simulink model "saved3"  (R2018b)
settings: Solver=VariableStepAuto  StartTime=0.0  StopTime=10.0  RelTol=1e-3
libraries: simulink x95, powerlib x8, powerlib_meascontrol x2
(part 1 of 6)
settings Model: Creator=71873  LastModifiedBy=71873

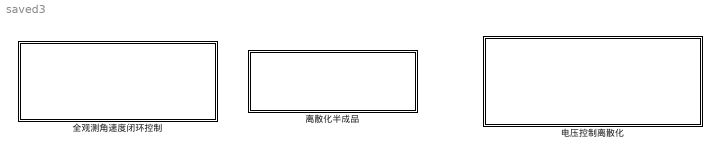
== system saved3 ==
  全观测角速度闭环控制 : Subsystem
  电压控制离散化 : Subsystem
  离散化半成品 : Subsystem

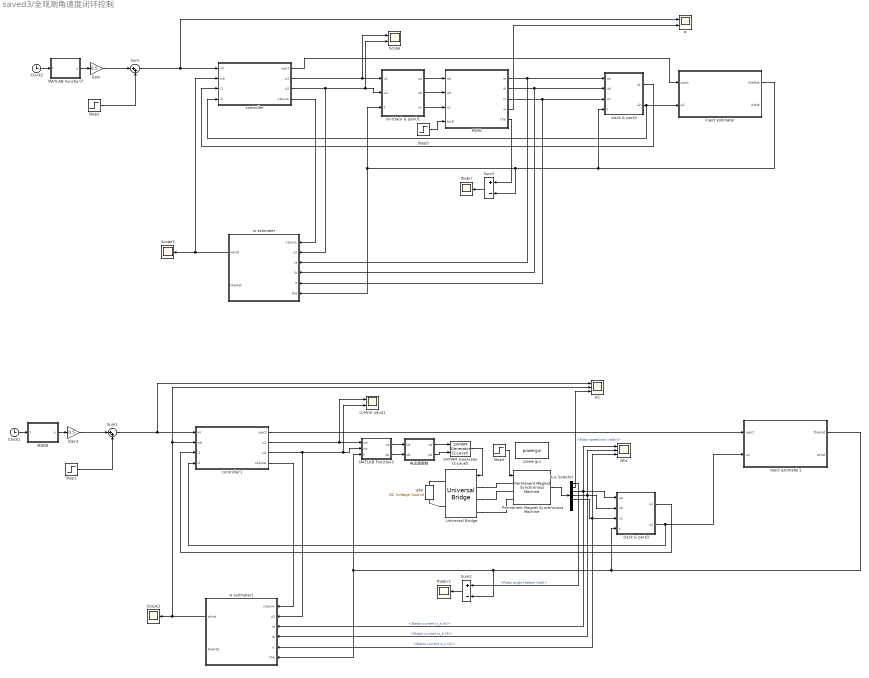
== system saved3/全观测角速度闭环控制 ==
  24V : powerlib/Electrical Sources/DC Voltage Source  Amplitude=24  Measurements=None
  Bus Selector : BusSelector  OutputSignals=Rotor angle thetam (rad),Rotor speed wm (rad/s),Stator current is_a (A),Stator current is_b (A),Stator current is_c (A),Stator current is_d (A),Stator current is_q (A)
  Clock1 : Clock
  Clock2 : Clock
  Gain : Gain  Gain=0.5
  Gain1 : Gain  Gain=0.5
  MATLAB Function3 : MATLAB Function  TreatAsAtomicUnit=on
  MATLAB Function7 : MATLAB Function  TreatAsAtomicUnit=on
  PSMS : Subsystem
  Permanent Magnet Synchronous Machine : powerlib/Machines/Permanent Magnet Synchronous Machine  NbPhases=3  FluxDistribution=Sinusoidal  RotorType=Salient-pole  MechanicalLoad=Torque Tm  PresetModel=No  ShowDetailedParameters=on  MeasurementBus=off  Resistance=0.1  Inductance=8.5e-3  dqInductances=[1e-3,1.4e-3]  La=0.000395  MachineConstant=Flux linkage established by magnets (V.s)  Flux=0.05  VoltageCst=9.069  TorqueCst=0.075  Flat=120  Mechanical=[1e-3 5e-4 1 0]  PolePairs=4  InitialConditions=[0,0, 0,0]  InitialConditions5ph=[0 0 0 0 0 0]  TsPowergui=0  TsBlock=-1  RefAngle=Aligned with phase A axis (original Park)
      settings: SourceProductName=Simscape Power Systems
  SVPWM Generator (2-Level) : powerlib_meascontrol/Pulse & Signal Generators/SVPWM Generator (2-Level)  InputType=alpha-beta components  SwitchingPattern=Pattern #1  Fc=20000  ParUref=[0.8 -30 50]  Ts=0
      settings: SourceProductName=Simscape Power Systems  SourceProductBaseCode=PS
  Scope : Scope  NumInputPorts=2
  Scope1 : Scope
  Scope3 : Scope
  Step1 : Step  Time=1.5  After=50  SampleTime=0
  Step2 : Step  Time=1.5  After=50  SampleTime=0
  Step3 : Step  After=0.5  SampleTime=0
  Step5 : Step  Time=0.8  After=0.25  SampleTime=0
  Sum : Sum  Inputs=|++
  Sum1 : Sum  Inputs=|++
  Sum2 : Sum  Inputs=+-
  Sum3 : Sum  Inputs=+-
  Universal Bridge : powerlib/Power Electronics/Universal Bridge  Arms=3  SnubberResistance=1e5  SnubberCapacitance=inf  Device=MOSFET / Diodes  Ron=1e-3  Lon=0  ForwardVoltages="[  0  0  ]"  ForwardVoltage=0  GTOparameters=[ 10e-6 , 20e-6 ]  IGBTparameters=[ 1e-6 , 2e-6 ]  Measurements=None  Measurements_2=None  converterType=Rectifier
  clack & park2 : MATLAB Function  TreatAsAtomicUnit=on
  clack & park3 : MATLAB Function  TreatAsAtomicUnit=on
  control uduq1 : Scope  NumInputPorts=2
  controller : Subsystem
  controller1 : Subsystem
  iabc : Scope  NumInputPorts=3
  inject estimater : Subsystem
  inject estimater1 : Subsystem
  inv(clack & park)1 : MATLAB Function  TreatAsAtomicUnit=on
  powergui : powerlib/powergui  Priority=1  SimulationMode=Discrete  SampleTime=1e-6  frequency=60  Iterations=50  frequencyindice=0  Pbase=100e6  ErrMax=1e-4  UnitsV=kV  UnitsW=MW  buscounter=0  FunctionMessages=off  echomessages=off  EnableUseOfTLC=off  CurrentSourceSwitches=off  DisableSnubberDevices=off  DisableRonSwitches=off  DisableVfSwitches=off  DisplayEquations=off  SolverType=Tustin/Backward Euler (TBE)  Interpol=off  ExternalGateDelay=off  methode=off  Ts=100  x0status=blocks  SPID=on  SwTol=0  HookPort=off  RestoreLinks=warning  ResistiveCurrentMeasurement=off  Frange=[0:2:500]  Ylog=off  Xlog=on  ShowGrid=off  save=off  variable=ZData  structure=0  ZoomFFT=off  StartTime=0.0  cycles=1  DisplayStyle=1  fundamental=60  FreqAxis=off  MaxFrequency=1000  frequencyindicesteady=1  RmsSteady=1  display=off
  theErr : Scope
  theErr1 : Scope
  w : Scope  NumInputPorts=2
  w estimater : Subsystem
  w estimater1 : Subsystem
  w1 : Scope  NumInputPorts=3
  电压圆限制 : MATLAB Function  TreatAsAtomicUnit=on
  软启动 : MATLAB Function  TreatAsAtomicUnit=on
  wires:
  controller/3(u2) -> inv(clack & park)1/2(u2), Scope/2, w estimater/2(u2)
  controller/2(u1) -> Scope/1, inv(clack & park)1/1(u1)
  Clock2/1 -> MATLAB Function7/1(t)
  inv(clack & park)1/2(ub) -> PSMS/2(ub)
  PSMS/2(ib) -> clack & park2/2(ub), w estimater/4(ib)
  Gain/1 -> Sum/1
  controller/4(u1pure) -> w estimater/1(u1pure)
  PSMS/5(the) -> Sum3/1
  MATLAB Function7/1(y) -> Gain/1
  Sum3/1 -> theErr/1
  PSMS/3(ic) -> clack & park2/3(uc), w estimater/5(ic)
  Step3/1 -> PSMS/4(torE)
  clack & park2/1(u1) -> controller/3(i1)
  PSMS/4(w) -> w/2
  inject estimater/1(theHat) -> inv(clack & park)1/3(t), w estimater/6(the), Sum3/2, clack & park2/4(t)
  inv(clack & park)1/3(uc) -> PSMS/3(uc)
  controller/1(uject) -> inject estimater/1(uject)
  w estimater/1(wHat) -> controller/2(wb), Scope3/1
  Sum/1 -> w/1, controller/1(wr)
  clack & park2/2(u2) -> controller/4(i2), inject estimater/2(u2)
  Step2/1 -> Sum/2
  inv(clack & park)1/1(ua) -> PSMS/1(ua)
  PSMS/1(ia) -> clack & park2/1(ua), w estimater/3(ia)
  controller1/4(u1pure) -> w estimater1/1(u1pure)
  Clock1/1 -> 软启动/1(t)
  Sum2/1 -> theErr1/1
  controller1/1(uject) -> inject estimater1/1(uject)
  clack & park3/1(u1) -> controller1/3(i1)
  SVPWM Generator (2-Level)/1 -> Universal Bridge/1
  clack & park3/2(u2) -> inject estimater1/2(u2), controller1/4(i2)
  Bus Selector/1 -> Sum2/1  "<Rotor angle thetam (rad)>"
  Bus Selector/4 -> w estimater1/4(ib), iabc/2, clack & park3/2(ub)  "<Stator current is_b (A)>"
  软启动/1(y) -> Gain1/1
  Permanent Magnet Synchronous Machine/1 -> Bus Selector/1
  MATLAB Function3/2(ub) -> 电压圆限制/2(Ub)
  Step5/1 -> Permanent Magnet Synchronous Machine/1
  inject estimater1/1(theHat) -> clack & park3/4(t), MATLAB Function3/3(t), w estimater1/6(the), Sum2/2
  Bus Selector/3 -> w estimater1/3(ia), iabc/1, clack & park3/1(ua)  "<Stator current is_a (A)>"
  controller1/2(u1) -> MATLAB Function3/1(ud), control uduq1/1
  MATLAB Function3/1(ua) -> 电压圆限制/1(Ua)
  电压圆限制/2(ub) -> SVPWM Generator (2-Level)/2
  controller1/3(u2) -> MATLAB Function3/2(uq), control uduq1/2, w estimater1/2(u2)
  Step1/1 -> Sum1/2
  电压圆限制/1(ua) -> SVPWM Generator (2-Level)/1
  w estimater1/1(wHat) -> w1/2, controller1/2(wb), Scope1/1
  Bus Selector/5 -> w estimater1/5(ic), iabc/3, clack & park3/3(uc)  "<Stator current is_c (A)>"
  Gain1/1 -> Sum1/1
  Bus Selector/2 -> w1/3  "<Rotor speed wm (rad/s)>"
  Sum1/1 -> w1/1, controller1/1(wr)
  connections:
  Universal Bridge/LConn3 -- Permanent Magnet Synchronous Machine/LConn3
  Universal Bridge/RConn1 -- 24V/RConn1
  Universal Bridge/RConn2 -- 24V/LConn1
  Universal Bridge/LConn2 -- Permanent Magnet Synchronous Machine/LConn2
  Universal Bridge/LConn1 -- Permanent Magnet Synchronous Machine/LConn1

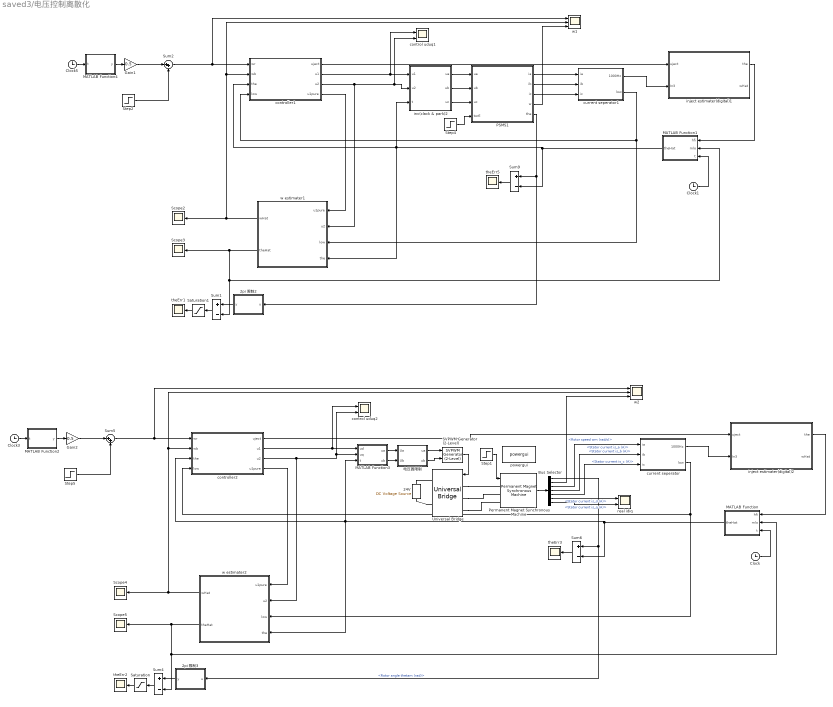
== system saved3/电压控制离散化 ==
  24V : powerlib/Electrical Sources/DC Voltage Source  Amplitude=24  Measurements=None
  2pi 限制2 : MATLAB Function  TreatAsAtomicUnit=on
  2pi 限制3 : MATLAB Function  TreatAsAtomicUnit=on
  Bus Selector : BusSelector  OutputSignals=Rotor angle thetam (rad),Rotor speed wm (rad/s),Stator current is_a (A),Stator current is_b (A),Stator current is_c (A),Stator current is_d (A),Stator current is_q (A)
  Clock{,1,3,5} (4 alike) : Clock
  Gain1 : Gain  Gain=0.5
  Gain2 : Gain  Gain=0.5
  MATLAB Function : MATLAB Function  TreatAsAtomicUnit=on
  MATLAB Function1 : MATLAB Function  TreatAsAtomicUnit=on
  MATLAB Function2 : MATLAB Function  TreatAsAtomicUnit=on
  MATLAB Function3 : MATLAB Function  TreatAsAtomicUnit=on
  MATLAB Function4 : MATLAB Function  TreatAsAtomicUnit=on
  PSMS1 : Subsystem
  Permanent Magnet Synchronous Machine : powerlib/Machines/Permanent Magnet Synchronous Machine  NbPhases=3  FluxDistribution=Sinusoidal  RotorType=Salient-pole  MechanicalLoad=Torque Tm  PresetModel=No  ShowDetailedParameters=on  MeasurementBus=off  Resistance=0.1  Inductance=8.5e-3  dqInductances=[1e-3,1.4e-3]  La=0.000395  MachineConstant=Flux linkage established by magnets (V.s)  Flux=0.05  VoltageCst=9.069  TorqueCst=0.075  Flat=120  Mechanical=[1e-3 5e-4 1 0]  PolePairs=4  InitialConditions=[0,0, 0,0]  InitialConditions5ph=[0 0 0 0 0 0]  TsPowergui=0  TsBlock=-1  RefAngle=Aligned with phase A axis (original Park)
      settings: SourceProductName=Simscape Power Systems
  SVPWM Generator (2-Level) : powerlib_meascontrol/Pulse & Signal Generators/SVPWM Generator (2-Level)  InputType=alpha-beta components  SwitchingPattern=Pattern #1  Fc=20000  ParUref=[0.8 -30 50]  Ts=0
      settings: SourceProductName=Simscape Power Systems  SourceProductBaseCode=PS
  Saturation : Saturate  UpperLimit=1  LowerLimit=-1
  Saturation1 : Saturate  UpperLimit=1  LowerLimit=-1
  Scope{2..5} (4 alike) : Scope
  Step1 : Step  Time=0.8  After=0.25  SampleTime=0
  Step2 : Step  Time=2  After=50  SampleTime=0
  Step4 : Step  After=0.5  SampleTime=0
  Step5 : Step  Time=2  After=50  SampleTime=0
  Sum{1,4,6,9} (4 alike) : Sum  Inputs=+-
  Sum2 : Sum  Inputs=|++
  Sum5 : Sum  Inputs=|++
  Universal Bridge : powerlib/Power Electronics/Universal Bridge  Arms=3  SnubberResistance=1e5  SnubberCapacitance=inf  Device=MOSFET / Diodes  Ron=1e-3  Lon=0  ForwardVoltages="[  0  0  ]"  ForwardVoltage=0  GTOparameters=[ 10e-6 , 20e-6 ]  IGBTparameters=[ 1e-6 , 2e-6 ]  Measurements=None  Measurements_2=None  converterType=Rectifier
  control uduq1 : Scope  NumInputPorts=2
  control uduq2 : Scope  NumInputPorts=2
  controller1 : Subsystem
  controller2 : Subsystem
  current seperator : Subsystem
  current seperator1 : Subsystem
  inject estimater(digital)1 : Subsystem
  inject estimater(digital)2 : Subsystem
  inv(clack & park)2 : MATLAB Function  TreatAsAtomicUnit=on
  powergui : powerlib/powergui  Priority=1  SimulationMode=Discrete  SampleTime=1e-6  frequency=60  Iterations=50  frequencyindice=0  Pbase=100e6  ErrMax=1e-4  UnitsV=kV  UnitsW=MW  buscounter=0  FunctionMessages=off  echomessages=off  EnableUseOfTLC=off  CurrentSourceSwitches=off  DisableSnubberDevices=off  DisableRonSwitches=off  DisableVfSwitches=off  DisplayEquations=off  SolverType=Tustin/Backward Euler (TBE)  Interpol=off  ExternalGateDelay=off  methode=off  Ts=100  x0status=blocks  SPID=on  SwTol=0  HookPort=off  RestoreLinks=warning  ResistiveCurrentMeasurement=off  Frange=[0:2:500]  Ylog=off  Xlog=on  ShowGrid=off  save=off  variable=ZData  structure=0  ZoomFFT=off  StartTime=0.0  cycles=1  DisplayStyle=1  fundamental=60  FreqAxis=off  MaxFrequency=1000  frequencyindicesteady=1  RmsSteady=1  display=off
  real idiq : Scope  NumInputPorts=2
  theErr{1..3,5} (4 alike) : Scope
  w estimater1 : Subsystem
  w estimater2 : Subsystem
  w1 : Scope  NumInputPorts=3
  w2 : Scope  NumInputPorts=3
  电压圆限制 : MATLAB Function  TreatAsAtomicUnit=on
  wires:
  controller2/2(u1) -> MATLAB Function3/1(ud), control uduq2/1
  电压圆限制/1(ua) -> SVPWM Generator (2-Level)/1
  w estimater2/1(wHat) -> Scope4/1, w2/2, controller2/2(wb)
  Bus Selector/6 -> real idiq/1  "<Stator current is_d (A)>"
  Clock3/1 -> MATLAB Function2/1(t)
  MATLAB Function2/1(y) -> Gain2/1
  Gain2/1 -> Sum5/1
  Saturation/1 -> theErr2/1
  w estimater2/2(theHat) -> Sum4/2, MATLAB Function/2(mlo), Scope5/1
  Sum4/1 -> Saturation/1
  Step1/1 -> Permanent Magnet Synchronous Machine/1
  Clock/1 -> MATLAB Function/3(t)
  Sum5/1 -> w2/1, controller2/1(wr)
  Step5/1 -> Sum5/2
  Bus Selector/5 -> current seperator/3(ic)  "<Stator current is_c (A)>"
  MATLAB Function3/2(ub) -> 电压圆限制/2(Ub)
  2pi 限制3/1(y) -> Sum4/1
  MATLAB Function/1(theHat) -> controller2/3(the), w estimater2/4(the), MATLAB Function3/3(t), Sum6/2
  Sum6/1 -> theErr3/1
  Permanent Magnet Synchronous Machine/1 -> Bus Selector/1
  MATLAB Function3/1(ua) -> 电压圆限制/1(Ua)
  controller2/4(u1pure) -> w estimater2/1(u1pure)
  Bus Selector/2 -> w2/3  "<Rotor speed wm (rad/s)>"
  inject estimater(digital)2/1(the) -> MATLAB Function/1(hfi)
  Bus Selector/4 -> current seperator/2(ib)  "<Stator current is_b (A)>"
  controller2/1(uject) -> inject estimater(digital)2/1(uject)
  controller2/3(u2) -> MATLAB Function3/2(uq), control uduq2/2, w estimater2/2(u2)
  Bus Selector/1 -> 2pi 限制3/1(u), Sum6/1  "<Rotor angle thetam (rad)>"
  SVPWM Generator (2-Level)/1 -> Universal Bridge/1
  电压圆限制/2(ub) -> SVPWM Generator (2-Level)/2
  Bus Selector/7 -> real idiq/2  "<Stator current is_q (A)>"
  current seperator/2(low) -> controller2/4(low), w estimater2/3(low)
  current seperator/1(1000Hz) -> inject estimater(digital)2/2(In3)
  Bus Selector/3 -> current seperator/1(ia)  "<Stator current is_a (A)>"
  controller1/3(u2) -> inv(clack & park)2/2(u2), control uduq1/2, w estimater1/2(u2)
  inv(clack & park)2/3(uc) -> PSMS1/3(uc)
  current seperator1/2(low) -> w estimater1/3(low), controller1/4(low)
  w estimater1/2(theHat) -> Sum1/2, MATLAB Function1/2(mlo), Scope3/1
  2pi 限制2/1(y) -> Sum1/1
  PSMS1/1(ia) -> current seperator1/1(ia)
  Sum1/1 -> Saturation1/1
  MATLAB Function1/1(theHat) -> inv(clack & park)2/3(t), controller1/3(the), w estimater1/4(the), Sum9/2
  Sum9/1 -> theErr5/1
  PSMS1/4(w) -> w1/3
  controller1/4(u1pure) -> w estimater1/1(u1pure)
  controller1/2(u1) -> control uduq1/1, inv(clack & park)2/1(u1)
  inject estimater(digital)1/1(the) -> MATLAB Function1/1(hfi)
  PSMS1/2(ib) -> current seperator1/2(ib)
  current seperator1/1(1000Hz) -> inject estimater(digital)1/2(In3)
  PSMS1/3(ic) -> current seperator1/3(ic)
  w estimater1/1(wHat) -> Scope2/1, w1/2, controller1/2(wb)
  Saturation1/1 -> theErr1/1
  Gain1/1 -> Sum2/1
  Step2/1 -> Sum2/2
  inv(clack & park)2/1(ua) -> PSMS1/1(ua)
  PSMS1/5(the) -> 2pi 限制2/1(u), Sum9/1
  Clock1/1 -> MATLAB Function1/3(t)
  inv(clack & park)2/2(ub) -> PSMS1/2(ub)
  Clock5/1 -> MATLAB Function4/1(t)
  MATLAB Function4/1(y) -> Gain1/1
  Step4/1 -> PSMS1/4(torE)
  controller1/1(uject) -> inject estimater(digital)1/1(uject)
  Sum2/1 -> w1/1, controller1/1(wr)
  connections:
  Universal Bridge/LConn3 -- Permanent Magnet Synchronous Machine/LConn3
  Universal Bridge/RConn1 -- 24V/RConn1
  Universal Bridge/LConn1 -- Permanent Magnet Synchronous Machine/LConn1
  Universal Bridge/RConn2 -- 24V/LConn1
  Universal Bridge/LConn2 -- Permanent Magnet Synchronous Machine/LConn2

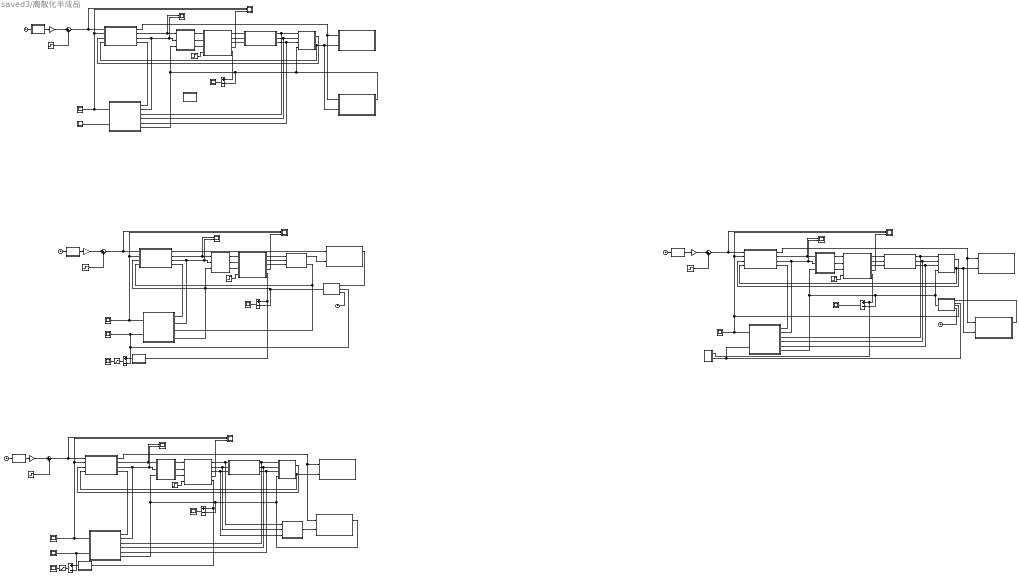
== system saved3/离散化半成品 ==
  2pi 限制1 : MATLAB Function  TreatAsAtomicUnit=on
  2pi 限制2 : MATLAB Function  TreatAsAtomicUnit=on
  2pi 限制3 : MATLAB Function  TreatAsAtomicUnit=on
  Clock{,1..5} (6 alike) : Clock
  Gain{,1..3} (4 alike) : Gain  Gain=0.5
  MATLAB Function : MATLAB Function  TreatAsAtomicUnit=on
  MATLAB Function1 : MATLAB Function  TreatAsAtomicUnit=on
  MATLAB Function2 : MATLAB Function  TreatAsAtomicUnit=on
  MATLAB Function3 : MATLAB Function  TreatAsAtomicUnit=on
  MATLAB Function4 : MATLAB Function  TreatAsAtomicUnit=on
  MATLAB Function7 : MATLAB Function  TreatAsAtomicUnit=on
  PSMS : Subsystem
  PSMS1 : Subsystem
  PSMS2 : Subsystem
  PSMS3 : Subsystem
  Saturation : Saturate  UpperLimit=1  LowerLimit=-1
  Saturation1 : Saturate  UpperLimit=1  LowerLimit=-1
  Scope{,1..6} (7 alike) : Scope
  Step1 : Step  Time=2  After=50  SampleTime=0
  Step2 : Step  Time=2  After=50  SampleTime=0
  Step{3..4,6,8} (4 alike) : Step  After=0.5  SampleTime=0
  Step5 : Step  Time=2  After=50  SampleTime=0
  Step7 : Step  Time=2  After=-50  SampleTime=0
  Subsystem : Subsystem
  Subsystem1 : Subsystem
  Sum{,2,5,7} (4 alike) : Sum  Inputs=|++
  Sum{1,3..4,6,8..9} (6 alike) : Sum  Inputs=+-
  clack & park1 : MATLAB Function  TreatAsAtomicUnit=on
  clack & park2 : MATLAB Function  TreatAsAtomicUnit=on
  clack & park3 : MATLAB Function  TreatAsAtomicUnit=on
  control uduq{,1..3} (4 alike) : Scope  NumInputPorts=2
  controller : Subsystem
  controller1 : Subsystem
  controller2 : Subsystem
  controller3 : Subsystem
  current seperator : Subsystem
  inject estimater : Subsystem
  inject estimater(digital) : Subsystem
  inject estimater(digital)1 : Subsystem
  inject estimater(digital)2 : Subsystem
  inject estimater(digital)3 : Subsystem
  inject estimater1 : Subsystem
  inject estimater2 : Subsystem
  inv(clack & park)1 : MATLAB Function  TreatAsAtomicUnit=on
  inv(clack & park)2 : MATLAB Function  TreatAsAtomicUnit=on
  inv(clack & park)3 : MATLAB Function  TreatAsAtomicUnit=on
  inv(clack & park)4 : MATLAB Function  TreatAsAtomicUnit=on
  theErr{,1..5} (6 alike) : Scope
  w{,1..3} (4 alike) : Scope  NumInputPorts=3
  w estimater : Subsystem
  w estimater1 : Subsystem
  w estimater2 : Subsystem
  w estimater3 : Subsystem
  电流采样 : Subsystem
  电流采样1 : Subsystem
  电流采样2 : Subsystem
  wires:
  controller/3(u2) -> inv(clack & park)1/2(u2), control uduq/2, w estimater/2(u2)
  inv(clack & park)1/1(ua) -> PSMS/1(ua)
  电流采样/2(ib) -> clack & park2/2(ub), w estimater/4(ib)
  PSMS/1(ia) -> 电流采样/1(<Stator current is_a (A)>)
  clack & park2/2(u2) -> inject estimater/2(u2), inject estimater(digital)/2(u2), controller/4(i2)
  inject estimater(digital)/1(theHat) -> Sum3/2, inv(clack & park)1/3(t), w estimater/6(the), clack & park2/4(t)
  PSMS/5(the) -> Sum3/1
  电流采样/3(ic) -> clack & park2/3(uc), w estimater/5(ic)
  Step3/1 -> PSMS/4(torE)
  inv(clack & park)1/2(ub) -> PSMS/2(ub)
  Sum/1 -> w/1, controller/1(wr)
  controller/1(uject) -> inject estimater/1(uject), inject estimater(digital)/1(uject)
  MATLAB Function7/1(y) -> Gain/1
  w estimater/1(wHat) -> Scope/1, w/2, controller/2(wb)
  PSMS/3(ic) -> 电流采样/3(<Stator current is_c (A)>)
  controller/4(u1pure) -> w estimater/1(u1pure)
  Sum3/1 -> theErr/1
  Gain/1 -> Sum/1
  Step2/1 -> Sum/2
  controller/2(u1) -> control uduq/1, inv(clack & park)1/1(u1)
  PSMS/2(ib) -> 电流采样/2(<Stator current is_b (A)>)
  clack & park2/1(u1) -> controller/3(i1)
  inv(clack & park)1/3(uc) -> PSMS/3(uc)
  电流采样/1(ia) -> clack & park2/1(ua), w estimater/3(ia)
  Clock2/1 -> MATLAB Function7/1(t)
  w estimater/2(theHat) -> Scope1/1
  PSMS/4(w) -> w/3
  PSMS2/4(w) -> w2/3
  controller2/2(u1) -> control uduq2/1, inv(clack & park)3/1(u1)
  inv(clack & park)3/2(ub) -> PSMS2/2(ub)
  inv(clack & park)3/1(ua) -> PSMS2/1(ua)
  PSMS2/3(ic) -> Subsystem/3(ic), 电流采样1/3(<Stator current is_c (A)>)
  controller2/4(u1pure) -> w estimater2/1(u1pure)
  inject estimater(digital)2/1(the) -> Sum6/2, inv(clack & park)3/3(t), w estimater2/6(the), clack & park1/4(t)
  电流采样1/1(ia) -> clack & park1/1(ua), w estimater2/3(ia)
  PSMS2/5(the) -> 2pi 限制3/1(u), Sum6/1
  电流采样1/2(ib) -> clack & park1/2(ub), w estimater2/4(ib)
  clack & park1/1(u1) -> controller2/3(i1)
  clack & park1/2(u2) -> inject estimater1/2(u2), controller2/4(i2)
  Sum5/1 -> w2/1, controller2/1(wr)
  PSMS2/1(ia) -> Subsystem/1(ia), 电流采样1/1(<Stator current is_a (A)>)
  PSMS2/2(ib) -> Subsystem/2(ib), 电流采样1/2(<Stator current is_b (A)>)
  Step6/1 -> PSMS2/4(torE)
  电流采样1/3(ic) -> clack & park1/3(uc), w estimater2/5(ic)
  Clock3/1 -> MATLAB Function2/1(t)
  Step5/1 -> Sum5/2
  inv(clack & park)3/3(uc) -> PSMS2/3(uc)
  Subsystem/1(1000Hz) -> inject estimater(digital)2/2(In3)
  Sum6/1 -> theErr3/1
  w estimater2/1(wHat) -> Scope4/1, w2/2, controller2/2(wb)
  Gain2/1 -> Sum5/1
  controller2/1(uject) -> inject estimater1/1(uject), inject estimater(digital)2/1(uject)
  w estimater2/2(theHat) -> Sum4/2, Scope5/1
  MATLAB Function2/1(y) -> Gain2/1
  Saturation/1 -> theErr2/1
  Sum4/1 -> Saturation/1
  controller2/3(u2) -> inv(clack & park)3/2(u2), control uduq2/2, w estimater2/2(u2)
  2pi 限制3/1(y) -> Sum4/1
  MATLAB Function/1(theHat) -> clack & park3/4(t), Sum8/2, inv(clack & park)4/3(t), w estimater3/6(the)
  inv(clack & park)4/3(uc) -> PSMS3/3(uc)
  Sum8/1 -> theErr4/1
  Sum7/1 -> w3/1, controller3/1(wr)
  PSMS3/4(w) -> w3/3
  Step7/1 -> Sum7/2
  controller3/3(u2) -> inv(clack & park)4/2(u2), control uduq3/2, w estimater3/2(u2)
  controller3/2(u1) -> control uduq3/1, inv(clack & park)4/1(u1)
  PSMS3/3(ic) -> 电流采样2/3(<Stator current is_c (A)>)
  controller3/4(u1pure) -> w estimater3/1(u1pure)
  clack & park3/1(u1) -> controller3/3(i1)
  inv(clack & park)4/1(ua) -> PSMS3/1(ua)
  电流采样2/2(ib) -> clack & park3/2(ub), w estimater3/4(ib)
  PSMS3/5(the) -> Subsystem1/1(ref), Sum8/1
  Clock/1 -> MATLAB Function/4(t)
  MATLAB Function3/1(y) -> Gain3/1
  电流采样2/3(ic) -> clack & park3/3(uc), w estimater3/5(ic)
  controller3/1(uject) -> inject estimater(digital)3/1(uject), inject estimater2/1(uject)
  PSMS3/1(ia) -> 电流采样2/1(<Stator current is_a (A)>)
  inv(clack & park)4/2(ub) -> PSMS3/2(ub)
  inject estimater(digital)3/1(theHat) -> MATLAB Function/1(Inj)
  电流采样2/1(ia) -> clack & park3/1(ua), w estimater3/3(ia)
  Clock4/1 -> MATLAB Function3/1(t)
  Gain3/1 -> Sum7/1
  PSMS3/2(ib) -> 电流采样2/2(<Stator current is_b (A)>)
  w estimater3/2(theHat) -> Subsystem1/2(in), MATLAB Function/2(Emf)
  Step8/1 -> PSMS3/4(torE)
  clack & park3/2(u2) -> inject estimater(digital)3/2(u2), inject estimater2/2(u2), controller3/4(i2)
  w estimater3/1(wHat) -> w3/2, controller3/2(wb), MATLAB Function/3(wHat), Scope6/1
  Clock1/1 -> MATLAB Function1/3(t)
  inv(clack & park)2/2(ub) -> PSMS1/2(ub)
  Sum2/1 -> w1/1, controller1/1(wr)
  MATLAB Function4/1(y) -> Gain1/1
  PSMS1/5(the) -> 2pi 限制2/1(u), Sum9/1
  Step1/1 -> Sum2/2
  PSMS1/3(ic) -> current seperator/3(ic)
  Gain1/1 -> Sum2/1
  Step4/1 -> PSMS1/4(torE)
  inv(clack & park)2/1(ua) -> PSMS1/1(ua)
  PSMS1/2(ib) -> current seperator/2(ib)
  controller1/1(uject) -> inject estimater(digital)1/1(uject)
  current seperator/1(1000Hz) -> inject estimater(digital)1/2(In3)
  controller1/2(u1) -> control uduq1/1, inv(clack & park)2/1(u1)
  inject estimater(digital)1/1(the) -> MATLAB Function1/1(hfi)
  controller1/4(u1pure) -> w estimater1/1(u1pure)
  Sum9/1 -> theErr5/1
  PSMS1/4(w) -> w1/3
  w estimater1/1(wHat) -> Scope2/1, w1/2, controller1/2(wb)
  Sum1/1 -> Saturation1/1
  2pi 限制2/1(y) -> Sum1/1
  MATLAB Function1/1(theHat) -> inv(clack & park)2/3(t), controller1/3(the), w estimater1/4(the), Sum9/2
  PSMS1/1(ia) -> current seperator/1(ia)
  Clock5/1 -> MATLAB Function4/1(t)
  current seperator/2(low) -> w estimater1/3(low), controller1/4(low)
  Saturation1/1 -> theErr1/1
  w estimater1/2(theHat) -> Sum1/2, MATLAB Function1/2(mlo), Scope3/1
  controller1/3(u2) -> inv(clack & park)2/2(u2), control uduq1/2, w estimater1/2(u2)
  inv(clack & park)2/3(uc) -> PSMS1/3(uc)

== system saved3/全观测角速度闭环控制/PSMS ==
  ua : Inport
  ub : Inport  Port=2
  uc : Inport  Port=3
  torE : Inport  Port=4
  PMSM dq : Subsystem
  clack & park : MATLAB Function  TreatAsAtomicUnit=on
  inv(clack & park) : MATLAB Function  TreatAsAtomicUnit=on
  ia : Outport
  ib : Outport  Port=2
  ic : Outport  Port=3
  w : Outport  Port=4
  the : Outport  Port=5
  wires:
  ua/1 -> clack & park/1(ua)
  PMSM dq/3(w) -> w/1
  PMSM dq/2(i2) -> inv(clack & park)/2(u2)
  torE/1 -> PMSM dq/3(torE)
  PMSM dq/4(the) -> inv(clack & park)/3(t), clack & park/4(t), the/1
  clack & park/1(u1) -> PMSM dq/1(u1)
  PMSM dq/1(i1) -> inv(clack & park)/1(u1)
  clack & park/2(u2) -> PMSM dq/2(u2)
  ub/1 -> clack & park/2(ub)
  uc/1 -> clack & park/3(uc)
  inv(clack & park)/1(ua) -> ia/1
  inv(clack & park)/3(uc) -> ic/1
  inv(clack & park)/2(ub) -> ib/1

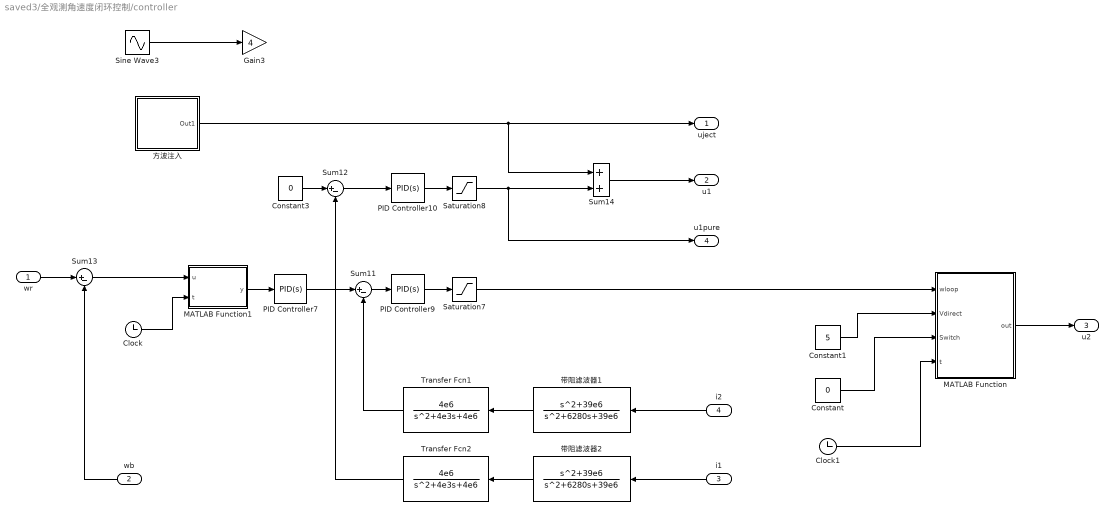
== system saved3/全观测角速度闭环控制/controller ==
  wr : Inport
  wb : Inport  Port=2
  i1 : Inport  Port=3
  i2 : Inport  Port=4
  Clock : Clock
  Clock1 : Clock
  Constant : Constant  Value=0
  Constant1 : Constant  Value=5
  Constant3 : Constant  Value=0
  Gain3 : Gain  Gain=4
  MATLAB Function : MATLAB Function  TreatAsAtomicUnit=on
  MATLAB Function1 : MATLAB Function  TreatAsAtomicUnit=on
  PID Controller10 : simulink/Continuous/PID Controller  Controller=PID  Form=Parallel  TimeDomain=Continuous-time  SampleTime=-1  IntegratorMethod=Forward Euler  FilterMethod=Forward Euler  ControllerParametersSource=internal  P=3  I=10  D=0  UseFilter=on  N=100  TunerSelectOption=Transfer Function Based (PID Tuner App)  InitialConditionSource=internal  InitialConditionForIntegrator=0  InitialConditionForFilter=0  DifferentiatorICPrevScaledInput=0  ExternalReset=none  TrackingMode=off  Kt=1  LimitOutput=off  UpperSaturationLimit=inf  LowerSaturationLimit=-inf  LinearizeAsGain=on  AntiWindupMode=none  Kb=1  POutMin=[]  POutMax=[]  IOutMin=[]  IOutMax=[]  DOutMin=[]  DOutMax=[]  NOutMin=[]  NOutMax=[]  SumOutMin=[]  SumOutMax=[]  SaturationOutMin=[]  SaturationOutMax=[]  PParamMin=[]  PParamMax=[]  IParamMin=[]  IParamMax=[]  DParamMin=[]  DParamMax=[]  NParamMin=[]  NParamMax=[]  KbParamMin=[]  KbParamMax=[]  KtParamMin=[]  KtParamMax=[]  KbOutMin=[]  KbOutMax=[]  KtOutMin=[]  KtOutMax=[]  IntegratorOutMin=[]  IntegratorOutMax=[]  FilterOutMin=[]  FilterOutMax=[]  SumI1OutMin=[]  SumI1OutMax=[]  SumI2OutMin=[]  SumI2OutMax=[]  SumI3OutMin=[]  SumI3OutMax=[]  SumI4OutMin=[]  SumI4OutMax=[]  SumDOutMin=[]  SumDOutMax=[]  DifferentiatorOutMin=[]  DifferentiatorOutMax=[]  FilterDiffOutCoefMin=[]  FilterDiffOutCoefMax=[]  ReciprocalOutMin=[]  ReciprocalOutMax=[]  SumDenOutMin=[]  SumDenOutMax=[]  SumNumOutMin=[]  SumNumOutMax=[]  DivideOutMin=[]  DivideOutMax=[]  IntegratorContinuousStateAttributes=''  IntegratorStateMustResolveToSignalObject=off  IntegratorRTWStateStorageClass=Auto  FilterContinuousStateAttributes=''  FilterStateMustResolveToSignalObject=off  FilterRTWStateStorageClass=Auto  ParallelPVariant=InternalParameters  IdealPVariant=Disabled  IVariant=InternalParameters  DVariant=InternalParameters  IntegratorVariant=Continuous  SatVariant=Disabled  AWVariant=Passthrough  PCopyVariant=Disabled  TRVariant=Disabled  FdbkBlocksVariant=Forward  IdealPFdbkVariant=Disabled  SatFdbkVariant=Disabled  DerivativeFilterVariant=ContFilter  NVariant=InternalParameters  NCopyVariant=Disabled  FilterICVariant=InternalICsFilter  IntegratorICVariant=InternalICs  ExternalResetVariant=Disabled  TRSumVariant=Passthrough  SumFdbkVariant=Disabled  SumVariant=Sum_PID
  PID Controller7 : simulink/Continuous/PID Controller  Controller=PID  Form=Parallel  TimeDomain=Continuous-time  SampleTime=1e-4  IntegratorMethod=Forward Euler  FilterMethod=Forward Euler  ControllerParametersSource=internal  P=0.3  I=5  D=0  UseFilter=on  N=100  TunerSelectOption=Transfer Function Based (PID Tuner App)  InitialConditionSource=internal  InitialConditionForIntegrator=0  InitialConditionForFilter=0  DifferentiatorICPrevScaledInput=0  ExternalReset=none  TrackingMode=off  Kt=1  LimitOutput=off  UpperSaturationLimit=inf  LowerSaturationLimit=-inf  LinearizeAsGain=on  AntiWindupMode=none  Kb=1  POutMin=[]  POutMax=[]  IOutMin=[]  IOutMax=[]  DOutMin=[]  DOutMax=[]  NOutMin=[]  NOutMax=[]  SumOutMin=[]  SumOutMax=[]  SaturationOutMin=[]  SaturationOutMax=[]  PParamMin=[]  PParamMax=[]  IParamMin=[]  IParamMax=[]  DParamMin=[]  DParamMax=[]  NParamMin=[]  NParamMax=[]  KbParamMin=[]  KbParamMax=[]  KtParamMin=[]  KtParamMax=[]  KbOutMin=[]  KbOutMax=[]  KtOutMin=[]  KtOutMax=[]  IntegratorOutMin=[]  IntegratorOutMax=[]  FilterOutMin=[]  FilterOutMax=[]  SumI1OutMin=[]  SumI1OutMax=[]  SumI2OutMin=[]  SumI2OutMax=[]  SumI3OutMin=[]  SumI3OutMax=[]  SumI4OutMin=[]  SumI4OutMax=[]  SumDOutMin=[]  SumDOutMax=[]  DifferentiatorOutMin=[]  DifferentiatorOutMax=[]  FilterDiffOutCoefMin=[]  FilterDiffOutCoefMax=[]  ReciprocalOutMin=[]  ReciprocalOutMax=[]  SumDenOutMin=[]  SumDenOutMax=[]  SumNumOutMin=[]  SumNumOutMax=[]  DivideOutMin=[]  DivideOutMax=[]  IntegratorContinuousStateAttributes=''  IntegratorStateMustResolveToSignalObject=off  IntegratorRTWStateStorageClass=Auto  FilterContinuousStateAttributes=''  FilterStateMustResolveToSignalObject=off  FilterRTWStateStorageClass=Auto  ParallelPVariant=InternalParameters  IdealPVariant=Disabled  IVariant=InternalParameters  DVariant=InternalParameters  IntegratorVariant=Continuous  SatVariant=Disabled  AWVariant=Passthrough  PCopyVariant=Disabled  TRVariant=Disabled  FdbkBlocksVariant=Forward  IdealPFdbkVariant=Disabled  SatFdbkVariant=Disabled  DerivativeFilterVariant=ContFilter  NVariant=InternalParameters  NCopyVariant=Disabled  FilterICVariant=InternalICsFilter  IntegratorICVariant=InternalICs  ExternalResetVariant=Disabled  TRSumVariant=Passthrough  SumFdbkVariant=Disabled  SumVariant=Sum_PID
  PID Controller9 : simulink/Continuous/PID Controller  Controller=PID  Form=Parallel  TimeDomain=Continuous-time  SampleTime=-1  IntegratorMethod=Forward Euler  FilterMethod=Forward Euler  ControllerParametersSource=internal  P=3  I=10  D=0  UseFilter=on  N=100  TunerSelectOption=Transfer Function Based (PID Tuner App)  InitialConditionSource=internal  InitialConditionForIntegrator=0  InitialConditionForFilter=0  DifferentiatorICPrevScaledInput=0  ExternalReset=none  TrackingMode=off  Kt=1  LimitOutput=off  UpperSaturationLimit=inf  LowerSaturationLimit=-inf  LinearizeAsGain=on  AntiWindupMode=none  Kb=1  POutMin=[]  POutMax=[]  IOutMin=[]  IOutMax=[]  DOutMin=[]  DOutMax=[]  NOutMin=[]  NOutMax=[]  SumOutMin=[]  SumOutMax=[]  SaturationOutMin=[]  SaturationOutMax=[]  PParamMin=[]  PParamMax=[]  IParamMin=[]  IParamMax=[]  DParamMin=[]  DParamMax=[]  NParamMin=[]  NParamMax=[]  KbParamMin=[]  KbParamMax=[]  KtParamMin=[]  KtParamMax=[]  KbOutMin=[]  KbOutMax=[]  KtOutMin=[]  KtOutMax=[]  IntegratorOutMin=[]  IntegratorOutMax=[]  FilterOutMin=[]  FilterOutMax=[]  SumI1OutMin=[]  SumI1OutMax=[]  SumI2OutMin=[]  SumI2OutMax=[]  SumI3OutMin=[]  SumI3OutMax=[]  SumI4OutMin=[]  SumI4OutMax=[]  SumDOutMin=[]  SumDOutMax=[]  DifferentiatorOutMin=[]  DifferentiatorOutMax=[]  FilterDiffOutCoefMin=[]  FilterDiffOutCoefMax=[]  ReciprocalOutMin=[]  ReciprocalOutMax=[]  SumDenOutMin=[]  SumDenOutMax=[]  SumNumOutMin=[]  SumNumOutMax=[]  DivideOutMin=[]  DivideOutMax=[]  IntegratorContinuousStateAttributes=''  IntegratorStateMustResolveToSignalObject=off  IntegratorRTWStateStorageClass=Auto  FilterContinuousStateAttributes=''  FilterStateMustResolveToSignalObject=off  FilterRTWStateStorageClass=Auto  ParallelPVariant=InternalParameters  IdealPVariant=Disabled  IVariant=InternalParameters  DVariant=InternalParameters  IntegratorVariant=Continuous  SatVariant=Disabled  AWVariant=Passthrough  PCopyVariant=Disabled  TRVariant=Disabled  FdbkBlocksVariant=Forward  IdealPFdbkVariant=Disabled  SatFdbkVariant=Disabled  DerivativeFilterVariant=ContFilter  NVariant=InternalParameters  NCopyVariant=Disabled  FilterICVariant=InternalICsFilter  IntegratorICVariant=InternalICs  ExternalResetVariant=Disabled  TRSumVariant=Passthrough  SumFdbkVariant=Disabled  SumVariant=Sum_PID
  Saturation7 : Saturate  UpperLimit=20  LowerLimit=-20
  Saturation8 : Saturate  UpperLimit=20  LowerLimit=-20
  Sine Wave3 : Sin  Frequency=1000*2*pi  SampleTime=0
  Sum11 : Sum  Inputs=|+-
  Sum12 : Sum  Inputs=|+-
  Sum13 : Sum  Inputs=|+-
  Sum14 : Sum
  Transfer Fcn1 : TransferFcn  Numerator=[4e6]  Denominator=[1 4e3 4e6]
  Transfer Fcn2 : TransferFcn  Numerator=[4e6]  Denominator=[1 4e3 4e6]
  带阻滤波器1 : TransferFcn  Numerator=[1 0 39e6]  Denominator=[1 6280 39e6]
  带阻滤波器2 : TransferFcn  Numerator=[1 0 39e6]  Denominator=[1 6280 39e6]
  方波注入 : Subsystem
  uject : Outport
  u1 : Outport  Port=2
  u2 : Outport  Port=3
  u1pure : Outport  Port=4
  wires:
  Sum11/1 -> PID Controller9/1
  wb/1 -> Sum13/2
  Clock/1 -> MATLAB Function1/2(t)
  Saturation8/1 -> u1pure/1, Sum14/2
  MATLAB Function1/1(y) -> PID Controller7/1
  Sum13/1 -> MATLAB Function1/1(u)
  Constant3/1 -> Sum12/1
  PID Controller9/1 -> Saturation7/1
  Sum14/1 -> u1/1
  方波注入/1(Out1) -> uject/1, Sum14/1
  PID Controller7/1 -> Sum11/1
  Sum12/1 -> PID Controller10/1
  PID Controller10/1 -> Saturation8/1
  Sine Wave3/1 -> Gain3/1
  i2/1 -> 带阻滤波器1/1
  带阻滤波器2/1 -> Transfer Fcn2/1
  带阻滤波器1/1 -> Transfer Fcn1/1
  i1/1 -> 带阻滤波器2/1
  Saturation7/1 -> MATLAB Function/1(wloop)
  wr/1 -> Sum13/1
  Transfer Fcn1/1 -> Sum11/2
  Transfer Fcn2/1 -> Sum12/2
  MATLAB Function/1(out) -> u2/1
  Clock1/1 -> MATLAB Function/4(t)
  Constant/1 -> MATLAB Function/3(Switch)
  Constant1/1 -> MATLAB Function/2(Vdirect)

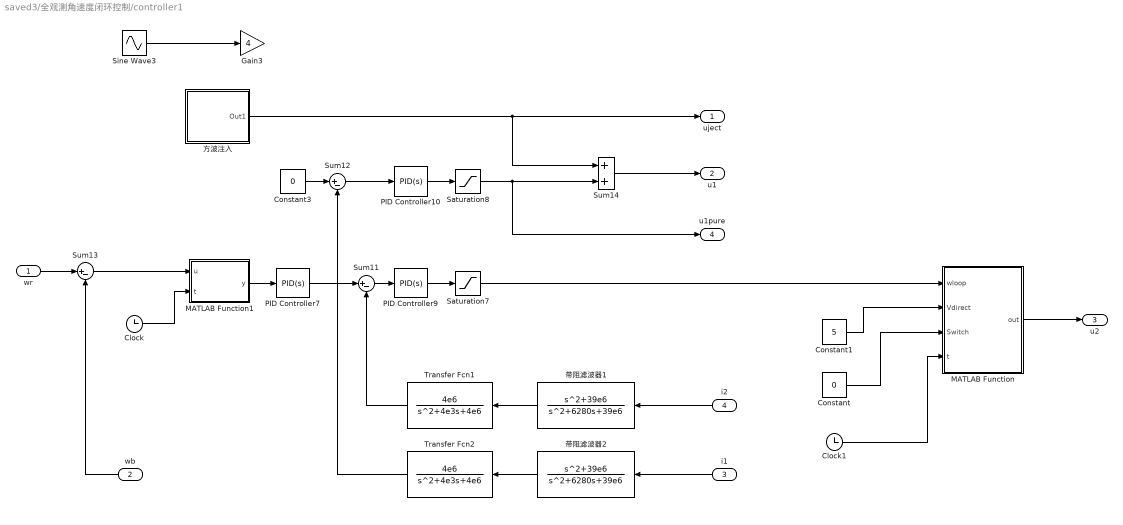
== system saved3/全观测角速度闭环控制/controller1 ==
  wr : Inport
  wb : Inport  Port=2
  i1 : Inport  Port=3
  i2 : Inport  Port=4
  Clock : Clock
  Clock1 : Clock
  Constant : Constant  Value=0
  Constant1 : Constant  Value=5
  Constant3 : Constant  Value=0
  Gain3 : Gain  Gain=4
  MATLAB Function : MATLAB Function  TreatAsAtomicUnit=on
  MATLAB Function1 : MATLAB Function  TreatAsAtomicUnit=on
  PID Controller10 : simulink/Continuous/PID Controller  Controller=PID  Form=Parallel  TimeDomain=Continuous-time  SampleTime=-1  IntegratorMethod=Forward Euler  FilterMethod=Forward Euler  ControllerParametersSource=internal  P=3  I=10  D=0  UseFilter=on  N=100  TunerSelectOption=Transfer Function Based (PID Tuner App)  InitialConditionSource=internal  InitialConditionForIntegrator=0  InitialConditionForFilter=0  DifferentiatorICPrevScaledInput=0  ExternalReset=none  TrackingMode=off  Kt=1  LimitOutput=off  UpperSaturationLimit=inf  LowerSaturationLimit=-inf  LinearizeAsGain=on  AntiWindupMode=none  Kb=1  POutMin=[]  POutMax=[]  IOutMin=[]  IOutMax=[]  DOutMin=[]  DOutMax=[]  NOutMin=[]  NOutMax=[]  SumOutMin=[]  SumOutMax=[]  SaturationOutMin=[]  SaturationOutMax=[]  PParamMin=[]  PParamMax=[]  IParamMin=[]  IParamMax=[]  DParamMin=[]  DParamMax=[]  NParamMin=[]  NParamMax=[]  KbParamMin=[]  KbParamMax=[]  KtParamMin=[]  KtParamMax=[]  KbOutMin=[]  KbOutMax=[]  KtOutMin=[]  KtOutMax=[]  IntegratorOutMin=[]  IntegratorOutMax=[]  FilterOutMin=[]  FilterOutMax=[]  SumI1OutMin=[]  SumI1OutMax=[]  SumI2OutMin=[]  SumI2OutMax=[]  SumI3OutMin=[]  SumI3OutMax=[]  SumI4OutMin=[]  SumI4OutMax=[]  SumDOutMin=[]  SumDOutMax=[]  DifferentiatorOutMin=[]  DifferentiatorOutMax=[]  FilterDiffOutCoefMin=[]  FilterDiffOutCoefMax=[]  ReciprocalOutMin=[]  ReciprocalOutMax=[]  SumDenOutMin=[]  SumDenOutMax=[]  SumNumOutMin=[]  SumNumOutMax=[]  DivideOutMin=[]  DivideOutMax=[]  IntegratorContinuousStateAttributes=''  IntegratorStateMustResolveToSignalObject=off  IntegratorRTWStateStorageClass=Auto  FilterContinuousStateAttributes=''  FilterStateMustResolveToSignalObject=off  FilterRTWStateStorageClass=Auto  ParallelPVariant=InternalParameters  IdealPVariant=Disabled  IVariant=InternalParameters  DVariant=InternalParameters  IntegratorVariant=Continuous  SatVariant=Disabled  AWVariant=Passthrough  PCopyVariant=Disabled  TRVariant=Disabled  FdbkBlocksVariant=Forward  IdealPFdbkVariant=Disabled  SatFdbkVariant=Disabled  DerivativeFilterVariant=ContFilter  NVariant=InternalParameters  NCopyVariant=Disabled  FilterICVariant=InternalICsFilter  IntegratorICVariant=InternalICs  ExternalResetVariant=Disabled  TRSumVariant=Passthrough  SumFdbkVariant=Disabled  SumVariant=Sum_PID
  PID Controller7 : simulink/Continuous/PID Controller  Controller=PID  Form=Parallel  TimeDomain=Continuous-time  SampleTime=1e-4  IntegratorMethod=Forward Euler  FilterMethod=Forward Euler  ControllerParametersSource=internal  P=0.3  I=5  D=0  UseFilter=on  N=100  TunerSelectOption=Transfer Function Based (PID Tuner App)  InitialConditionSource=internal  InitialConditionForIntegrator=0  InitialConditionForFilter=0  DifferentiatorICPrevScaledInput=0  ExternalReset=none  TrackingMode=off  Kt=1  LimitOutput=off  UpperSaturationLimit=inf  LowerSaturationLimit=-inf  LinearizeAsGain=on  AntiWindupMode=none  Kb=1  POutMin=[]  POutMax=[]  IOutMin=[]  IOutMax=[]  DOutMin=[]  DOutMax=[]  NOutMin=[]  NOutMax=[]  SumOutMin=[]  SumOutMax=[]  SaturationOutMin=[]  SaturationOutMax=[]  PParamMin=[]  PParamMax=[]  IParamMin=[]  IParamMax=[]  DParamMin=[]  DParamMax=[]  NParamMin=[]  NParamMax=[]  KbParamMin=[]  KbParamMax=[]  KtParamMin=[]  KtParamMax=[]  KbOutMin=[]  KbOutMax=[]  KtOutMin=[]  KtOutMax=[]  IntegratorOutMin=[]  IntegratorOutMax=[]  FilterOutMin=[]  FilterOutMax=[]  SumI1OutMin=[]  SumI1OutMax=[]  SumI2OutMin=[]  SumI2OutMax=[]  SumI3OutMin=[]  SumI3OutMax=[]  SumI4OutMin=[]  SumI4OutMax=[]  SumDOutMin=[]  SumDOutMax=[]  DifferentiatorOutMin=[]  DifferentiatorOutMax=[]  FilterDiffOutCoefMin=[]  FilterDiffOutCoefMax=[]  ReciprocalOutMin=[]  ReciprocalOutMax=[]  SumDenOutMin=[]  SumDenOutMax=[]  SumNumOutMin=[]  SumNumOutMax=[]  DivideOutMin=[]  DivideOutMax=[]  IntegratorContinuousStateAttributes=''  IntegratorStateMustResolveToSignalObject=off  IntegratorRTWStateStorageClass=Auto  FilterContinuousStateAttributes=''  FilterStateMustResolveToSignalObject=off  FilterRTWStateStorageClass=Auto  ParallelPVariant=InternalParameters  IdealPVariant=Disabled  IVariant=InternalParameters  DVariant=InternalParameters  IntegratorVariant=Continuous  SatVariant=Disabled  AWVariant=Passthrough  PCopyVariant=Disabled  TRVariant=Disabled  FdbkBlocksVariant=Forward  IdealPFdbkVariant=Disabled  SatFdbkVariant=Disabled  DerivativeFilterVariant=ContFilter  NVariant=InternalParameters  NCopyVariant=Disabled  FilterICVariant=InternalICsFilter  IntegratorICVariant=InternalICs  ExternalResetVariant=Disabled  TRSumVariant=Passthrough  SumFdbkVariant=Disabled  SumVariant=Sum_PID
  PID Controller9 : simulink/Continuous/PID Controller  Controller=PID  Form=Parallel  TimeDomain=Continuous-time  SampleTime=-1  IntegratorMethod=Forward Euler  FilterMethod=Forward Euler  ControllerParametersSource=internal  P=3  I=10  D=0  UseFilter=on  N=100  TunerSelectOption=Transfer Function Based (PID Tuner App)  InitialConditionSource=internal  InitialConditionForIntegrator=0  InitialConditionForFilter=0  DifferentiatorICPrevScaledInput=0  ExternalReset=none  TrackingMode=off  Kt=1  LimitOutput=off  UpperSaturationLimit=inf  LowerSaturationLimit=-inf  LinearizeAsGain=on  AntiWindupMode=none  Kb=1  POutMin=[]  POutMax=[]  IOutMin=[]  IOutMax=[]  DOutMin=[]  DOutMax=[]  NOutMin=[]  NOutMax=[]  SumOutMin=[]  SumOutMax=[]  SaturationOutMin=[]  SaturationOutMax=[]  PParamMin=[]  PParamMax=[]  IParamMin=[]  IParamMax=[]  DParamMin=[]  DParamMax=[]  NParamMin=[]  NParamMax=[]  KbParamMin=[]  KbParamMax=[]  KtParamMin=[]  KtParamMax=[]  KbOutMin=[]  KbOutMax=[]  KtOutMin=[]  KtOutMax=[]  IntegratorOutMin=[]  IntegratorOutMax=[]  FilterOutMin=[]  FilterOutMax=[]  SumI1OutMin=[]  SumI1OutMax=[]  SumI2OutMin=[]  SumI2OutMax=[]  SumI3OutMin=[]  SumI3OutMax=[]  SumI4OutMin=[]  SumI4OutMax=[]  SumDOutMin=[]  SumDOutMax=[]  DifferentiatorOutMin=[]  DifferentiatorOutMax=[]  FilterDiffOutCoefMin=[]  FilterDiffOutCoefMax=[]  ReciprocalOutMin=[]  ReciprocalOutMax=[]  SumDenOutMin=[]  SumDenOutMax=[]  SumNumOutMin=[]  SumNumOutMax=[]  DivideOutMin=[]  DivideOutMax=[]  IntegratorContinuousStateAttributes=''  IntegratorStateMustResolveToSignalObject=off  IntegratorRTWStateStorageClass=Auto  FilterContinuousStateAttributes=''  FilterStateMustResolveToSignalObject=off  FilterRTWStateStorageClass=Auto  ParallelPVariant=InternalParameters  IdealPVariant=Disabled  IVariant=InternalParameters  DVariant=InternalParameters  IntegratorVariant=Continuous  SatVariant=Disabled  AWVariant=Passthrough  PCopyVariant=Disabled  TRVariant=Disabled  FdbkBlocksVariant=Forward  IdealPFdbkVariant=Disabled  SatFdbkVariant=Disabled  DerivativeFilterVariant=ContFilter  NVariant=InternalParameters  NCopyVariant=Disabled  FilterICVariant=InternalICsFilter  IntegratorICVariant=InternalICs  ExternalResetVariant=Disabled  TRSumVariant=Passthrough  SumFdbkVariant=Disabled  SumVariant=Sum_PID
  Saturation7 : Saturate  UpperLimit=20  LowerLimit=-20
  Saturation8 : Saturate  UpperLimit=20  LowerLimit=-20
  Sine Wave3 : Sin  Frequency=1000*2*pi  SampleTime=0
  Sum11 : Sum  Inputs=|+-
  Sum12 : Sum  Inputs=|+-
  Sum13 : Sum  Inputs=|+-
  Sum14 : Sum
  Transfer Fcn1 : TransferFcn  Numerator=[4e6]  Denominator=[1 4e3 4e6]
  Transfer Fcn2 : TransferFcn  Numerator=[4e6]  Denominator=[1 4e3 4e6]
  带阻滤波器1 : TransferFcn  Numerator=[1 0 39e6]  Denominator=[1 6280 39e6]
  带阻滤波器2 : TransferFcn  Numerator=[1 0 39e6]  Denominator=[1 6280 39e6]
  方波注入 : Subsystem
  uject : Outport
  u1 : Outport  Port=2
  u2 : Outport  Port=3
  u1pure : Outport  Port=4
  wires:
  Sum11/1 -> PID Controller9/1
  wb/1 -> Sum13/2
  Clock/1 -> MATLAB Function1/2(t)
  Saturation8/1 -> u1pure/1, Sum14/2
  MATLAB Function1/1(y) -> PID Controller7/1
  Sum13/1 -> MATLAB Function1/1(u)
  Constant3/1 -> Sum12/1
  PID Controller9/1 -> Saturation7/1
  Sum14/1 -> u1/1
  方波注入/1(Out1) -> uject/1, Sum14/1
  PID Controller7/1 -> Sum11/1
  Sum12/1 -> PID Controller10/1
  PID Controller10/1 -> Saturation8/1
  Sine Wave3/1 -> Gain3/1
  i2/1 -> 带阻滤波器1/1
  带阻滤波器2/1 -> Transfer Fcn2/1
  带阻滤波器1/1 -> Transfer Fcn1/1
  i1/1 -> 带阻滤波器2/1
  Saturation7/1 -> MATLAB Function/1(wloop)
  wr/1 -> Sum13/1
  Transfer Fcn1/1 -> Sum11/2
  Transfer Fcn2/1 -> Sum12/2
  MATLAB Function/1(out) -> u2/1
  Clock1/1 -> MATLAB Function/4(t)
  Constant/1 -> MATLAB Function/3(Switch)
  Constant1/1 -> MATLAB Function/2(Vdirect)

== system saved3/全观测角速度闭环控制/inject estimater ==
  uject : Inport
  u2 : Inport  Port=2
  Gain6 : Gain  Gain=0.01
  Gain8 : Gain  Gain=-100
  Integrator2 : Integrator  InitialCondition=0.3
  PID Controller2 : simulink/Continuous/PID Controller  Controller=PID  Form=Parallel  TimeDomain=Continuous-time  SampleTime=-1  IntegratorMethod=Forward Euler  FilterMethod=Forward Euler  ControllerParametersSource=internal  P=4  I=350  D=0  UseFilter=on  N=100  TunerSelectOption=Transfer Function Based (PID Tuner App)  InitialConditionSource=internal  InitialConditionForIntegrator=0  InitialConditionForFilter=0  DifferentiatorICPrevScaledInput=0  ExternalReset=none  TrackingMode=off  Kt=1  LimitOutput=off  UpperSaturationLimit=inf  LowerSaturationLimit=-inf  LinearizeAsGain=on  AntiWindupMode=none  Kb=1  POutMin=[]  POutMax=[]  IOutMin=[]  IOutMax=[]  DOutMin=[]  DOutMax=[]  NOutMin=[]  NOutMax=[]  SumOutMin=[]  SumOutMax=[]  SaturationOutMin=[]  SaturationOutMax=[]  PParamMin=[]  PParamMax=[]  IParamMin=[]  IParamMax=[]  DParamMin=[]  DParamMax=[]  NParamMin=[]  NParamMax=[]  KbParamMin=[]  KbParamMax=[]  KtParamMin=[]  KtParamMax=[]  KbOutMin=[]  KbOutMax=[]  KtOutMin=[]  KtOutMax=[]  IntegratorOutMin=[]  IntegratorOutMax=[]  FilterOutMin=[]  FilterOutMax=[]  SumI1OutMin=[]  SumI1OutMax=[]  SumI2OutMin=[]  SumI2OutMax=[]  SumI3OutMin=[]  SumI3OutMax=[]  SumI4OutMin=[]  SumI4OutMax=[]  SumDOutMin=[]  SumDOutMax=[]  DifferentiatorOutMin=[]  DifferentiatorOutMax=[]  FilterDiffOutCoefMin=[]  FilterDiffOutCoefMax=[]  ReciprocalOutMin=[]  ReciprocalOutMax=[]  SumDenOutMin=[]  SumDenOutMax=[]  SumNumOutMin=[]  SumNumOutMax=[]  DivideOutMin=[]  DivideOutMax=[]  IntegratorContinuousStateAttributes=''  IntegratorStateMustResolveToSignalObject=off  IntegratorRTWStateStorageClass=Auto  FilterContinuousStateAttributes=''  FilterStateMustResolveToSignalObject=off  FilterRTWStateStorageClass=Auto  ParallelPVariant=InternalParameters  IdealPVariant=Disabled  IVariant=InternalParameters  DVariant=InternalParameters  IntegratorVariant=Continuous  SatVariant=Disabled  AWVariant=Passthrough  PCopyVariant=Disabled  TRVariant=Disabled  FdbkBlocksVariant=Forward  IdealPFdbkVariant=Disabled  SatFdbkVariant=Disabled  DerivativeFilterVariant=ContFilter  NVariant=InternalParameters  NCopyVariant=Disabled  FilterICVariant=InternalICsFilter  IntegratorICVariant=InternalICs  ExternalResetVariant=Disabled  TRSumVariant=Passthrough  SumFdbkVariant=Disabled  SumVariant=Sum_PID
  Ramp2 : simulink/Sources/Ramp  slope=0  start=0  InitialOutput=0
  Scope19 : Scope
  Scope7 : Scope  NumInputPorts=2
  Sum2 : Sum  Inputs=|++
  Transfer Fcn2 : TransferFcn  Numerator=[6280 0]  Denominator=[1 6280 39e6]
  低通滤波器 : TransferFcn  Numerator=[25e4]  Denominator=[1 500 25e4]
  带通滤波器1 : TransferFcn  Numerator=[6280 0]  Denominator=[1 6280 39e6]
  带通滤波器2 : TransferFcn  Numerator=[6280 0]  Denominator=[1 6280 39e6]
  混频 : Product
  相移器-90° : TransferFcn  Numerator=[39e6]  Denominator=[1 6280 39e6]
  theHat : Outport
  wHat : Outport  Port=2
  wires:
  相移器-90°/1 -> 混频/1
  混频/1 -> 低通滤波器/1
  Gain6/1 -> Scope7/1
  带通滤波器2/1 -> Transfer Fcn2/1
  Transfer Fcn2/1 -> 相移器-90°/1, Scope7/2
  PID Controller2/1 -> Sum2/1
  Integrator2/1 -> theHat/1
  Gain8/1 -> PID Controller2/1
  Ramp2/1 -> Sum2/2
  带通滤波器1/1 -> 混频/2, Gain6/1
  u2/1 -> 带通滤波器2/1
  uject/1 -> 带通滤波器1/1
  Sum2/1 -> wHat/1, Integrator2/1
  低通滤波器/1 -> Gain8/1, Scope19/1

== system saved3/全观测角速度闭环控制/inject estimater1 ==
  uject : Inport
  u2 : Inport  Port=2
  Gain6 : Gain  Gain=0.01
  Gain8 : Gain  Gain=-100
  Integrator2 : Integrator  InitialCondition=0.3
  PID Controller2 : simulink/Continuous/PID Controller  Controller=PID  Form=Parallel  TimeDomain=Continuous-time  SampleTime=-1  IntegratorMethod=Forward Euler  FilterMethod=Forward Euler  ControllerParametersSource=internal  P=4  I=350  D=0  UseFilter=on  N=100  TunerSelectOption=Transfer Function Based (PID Tuner App)  InitialConditionSource=internal  InitialConditionForIntegrator=0  InitialConditionForFilter=0  DifferentiatorICPrevScaledInput=0  ExternalReset=none  TrackingMode=off  Kt=1  LimitOutput=off  UpperSaturationLimit=inf  LowerSaturationLimit=-inf  LinearizeAsGain=on  AntiWindupMode=none  Kb=1  POutMin=[]  POutMax=[]  IOutMin=[]  IOutMax=[]  DOutMin=[]  DOutMax=[]  NOutMin=[]  NOutMax=[]  SumOutMin=[]  SumOutMax=[]  SaturationOutMin=[]  SaturationOutMax=[]  PParamMin=[]  PParamMax=[]  IParamMin=[]  IParamMax=[]  DParamMin=[]  DParamMax=[]  NParamMin=[]  NParamMax=[]  KbParamMin=[]  KbParamMax=[]  KtParamMin=[]  KtParamMax=[]  KbOutMin=[]  KbOutMax=[]  KtOutMin=[]  KtOutMax=[]  IntegratorOutMin=[]  IntegratorOutMax=[]  FilterOutMin=[]  FilterOutMax=[]  SumI1OutMin=[]  SumI1OutMax=[]  SumI2OutMin=[]  SumI2OutMax=[]  SumI3OutMin=[]  SumI3OutMax=[]  SumI4OutMin=[]  SumI4OutMax=[]  SumDOutMin=[]  SumDOutMax=[]  DifferentiatorOutMin=[]  DifferentiatorOutMax=[]  FilterDiffOutCoefMin=[]  FilterDiffOutCoefMax=[]  ReciprocalOutMin=[]  ReciprocalOutMax=[]  SumDenOutMin=[]  SumDenOutMax=[]  SumNumOutMin=[]  SumNumOutMax=[]  DivideOutMin=[]  DivideOutMax=[]  IntegratorContinuousStateAttributes=''  IntegratorStateMustResolveToSignalObject=off  IntegratorRTWStateStorageClass=Auto  FilterContinuousStateAttributes=''  FilterStateMustResolveToSignalObject=off  FilterRTWStateStorageClass=Auto  ParallelPVariant=InternalParameters  IdealPVariant=Disabled  IVariant=InternalParameters  DVariant=InternalParameters  IntegratorVariant=Continuous  SatVariant=Disabled  AWVariant=Passthrough  PCopyVariant=Disabled  TRVariant=Disabled  FdbkBlocksVariant=Forward  IdealPFdbkVariant=Disabled  SatFdbkVariant=Disabled  DerivativeFilterVariant=ContFilter  NVariant=InternalParameters  NCopyVariant=Disabled  FilterICVariant=InternalICsFilter  IntegratorICVariant=InternalICs  ExternalResetVariant=Disabled  TRSumVariant=Passthrough  SumFdbkVariant=Disabled  SumVariant=Sum_PID
  Ramp2 : simulink/Sources/Ramp  slope=0  start=0  InitialOutput=0
  Scope19 : Scope
  Scope7 : Scope  NumInputPorts=2
  Sum2 : Sum  Inputs=|++
  Transfer Fcn2 : TransferFcn  Numerator=[6280 0]  Denominator=[1 6280 39e6]
  低通滤波器 : TransferFcn  Numerator=[25e4]  Denominator=[1 500 25e4]
  带通滤波器1 : TransferFcn  Numerator=[6280 0]  Denominator=[1 6280 39e6]
  带通滤波器2 : TransferFcn  Numerator=[6280 0]  Denominator=[1 6280 39e6]
  混频 : Product
  相移器-90° : TransferFcn  Numerator=[39e6]  Denominator=[1 6280 39e6]
  theHat : Outport
  wHat : Outport  Port=2
  wires:
  相移器-90°/1 -> 混频/1
  混频/1 -> 低通滤波器/1
  Gain6/1 -> Scope7/1
  带通滤波器2/1 -> Transfer Fcn2/1
  Transfer Fcn2/1 -> 相移器-90°/1, Scope7/2
  PID Controller2/1 -> Sum2/1
  Integrator2/1 -> theHat/1
  Gain8/1 -> PID Controller2/1
  Ramp2/1 -> Sum2/2
  带通滤波器1/1 -> 混频/2, Gain6/1
  u2/1 -> 带通滤波器2/1
  uject/1 -> 带通滤波器1/1
  Sum2/1 -> wHat/1, Integrator2/1
  低通滤波器/1 -> Gain8/1, Scope19/1

== system saved3/全观测角速度闭环控制/w estimater ==
  u1pure : Inport
  u2 : Inport  Port=2
  ia : Inport  Port=3
  ib : Inport  Port=4
  ic : Inport  Port=5
  the : Inport  Port=6
  MATLAB Function : MATLAB Function  TreatAsAtomicUnit=on
  Subsystem : Subsystem
  Transfer Fcn : TransferFcn  Numerator=[4e6]  Denominator=[1 4e3 4e6]
  Transfer Fcn1 : TransferFcn  Numerator=[4e6]  Denominator=[1 4e3 4e6]
  clack : MATLAB Function  TreatAsAtomicUnit=on
  iabc : Scope  NumInputPorts=3
  invpark : MATLAB Function  TreatAsAtomicUnit=on
  带阻滤波器 : TransferFcn  Numerator=[1 0 39e6]  Denominator=[1 6280 39e6]
  带阻滤波器1 : TransferFcn  Numerator=[1 0 39e6]  Denominator=[1 6280 39e6]
  数据融合 : MATLAB Function  Commented=on  TreatAsAtomicUnit=on
  计算法求角速度 : MATLAB Function  Commented=on  TreatAsAtomicUnit=on
  锁相环 : Subsystem
  wHat : Outport
  theHat : Outport  Port=2
  wires:
  ib/1 -> clack/2(ib), iabc/2
  Subsystem/1(Ea) -> MATLAB Function/1(Ea), 锁相环/1(cos)
  Subsystem/2(Eb) -> MATLAB Function/2(Eb), 锁相环/2(sin)
  invpark/2(ub) -> Subsystem/2(ub)
  clack/1(iap) -> 带阻滤波器/1
  u2/1 -> invpark/2(u2)
  clack/2(ibe) -> 带阻滤波器1/1
  invpark/1(ua) -> Subsystem/1(ua)
  ia/1 -> clack/1(ia), iabc/1
  ic/1 -> clack/3(ic), iabc/3
  u1pure/1 -> invpark/1(u1)
  the/1 -> invpark/3(t)
  锁相环/1(we) -> wHat/1
  带阻滤波器1/1 -> Transfer Fcn/1
  带阻滤波器/1 -> Transfer Fcn1/1
  Transfer Fcn1/1 -> Subsystem/3(ia)
  Transfer Fcn/1 -> Subsystem/4(ib)
  MATLAB Function/1(y) -> theHat/1
